simulink model "DemoModel"  (R2019b)
settings: Solver=ode4  StartTime=0.0  StopTime=Inf  FixedStep=0.001  RelTol=1e-3
libraries: fl_lib x42, ElectricalElements x27, nesl_utility x5, simulink x3, ee_lib x2
settings Model: Creator=alfon  LastModifiedBy=Alfonso
settings SFSimCC: CustomCodeUndefinedFunction=UseInterfaceOnly

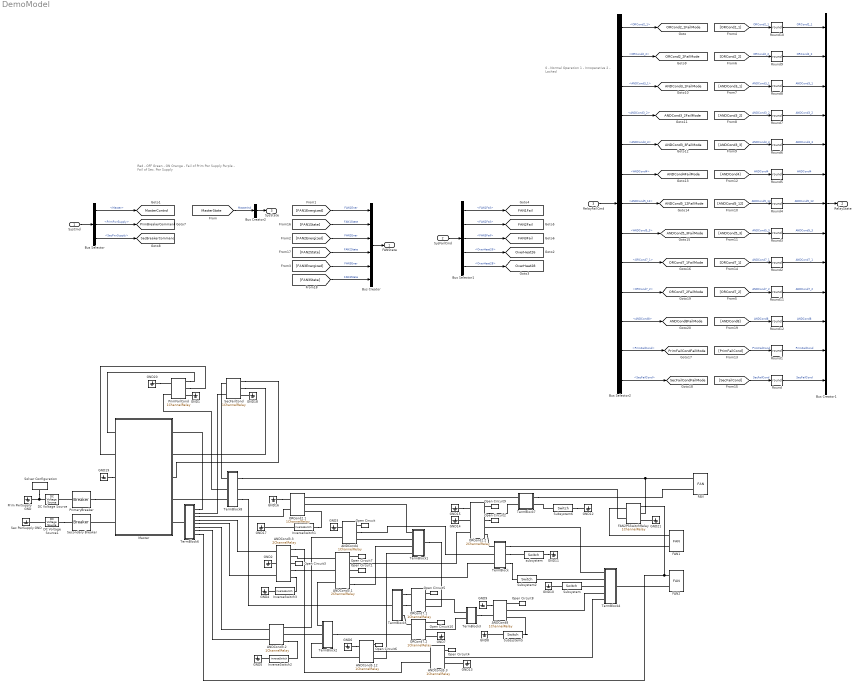
== system DemoModel ==
  note: Red - OFF
      | Green - ON
      | Orange - Fail of Prim Pwr Supply
      | Purple - Fail of Sec. Pwr Supply
  note: 0 - Normal Operation
      | 1 - Innoperative
      | 2 - Lached
  SysCmd : Inport  OutDataTypeStr=Bus: SysCmd  SampleTime=[0.001 0]
  SysFailCmd : Inport  Port=2  OutDataTypeStr=Bus: SysFailCmd  SampleTime=[0.001 0]
  RelayFailCmd : Inport  Port=3  OutDataTypeStr=Bus: RelayFailCmd  SampleTime=[0.001 0]
  ANDCond3.1 : ElectricalElements/Switches/2ChannelRelay  R=100  MinOpVolt=32  MaxOpVolt=22  RelayStateTag=ANDCond3_1  RelayFailModeTag=ANDCond3_1FailMode
  ANDCond3.2 : ElectricalElements/Switches/1ChannelRelay  R=100  MinOpVolt=32  MaxOpVolt=22  RelayStateTag=ANDCond3_2  RelayFailModeTag=ANDCond3_2FailMode
  ANDCond3.3 : ElectricalElements/Switches/2ChannelRelay  R=100  MinOpVolt=32  MaxOpVolt=22  RelayStateTag=ANDCond3_3  RelayFailModeTag=ANDCond3_3FailMode
  ANDCond4 : ElectricalElements/Switches/1ChannelRelay  R=100  MinOpVolt=32  MaxOpVolt=22  RelayStateTag=ANDCond4  RelayFailModeTag=ANDCond4FailMode
  ANDCond5.12 : ElectricalElements/Switches/1ChannelRelay  R=100  MinOpVolt=32  MaxOpVolt=22  RelayStateTag=ANDCond5_12  RelayFailModeTag=ANDCond5_12FailMode
  ANDCond5.3 : ElectricalElements/Switches/1ChannelRelay  R=100  MinOpVolt=32  MaxOpVolt=22  RelayStateTag=ANDCond5_3  RelayFailModeTag=ANDCond5_3FailMode
  ANDCond8 : ElectricalElements/Switches/1ChannelRelay  R=100  MinOpVolt=32  MaxOpVolt=22  RelayStateTag=ANDCond8  RelayFailModeTag=ANDCond8FailMode
  Bus Creator : BusCreator  Inputs=6
  Bus Creator1 : BusCreator  Inputs=13
  Bus Creator2 : BusCreator  Inputs=1
  Bus Selector : BusSelector  OutputSignals=Master,PrimPwrSupply,SecPwrSupply
  Bus Selector1 : BusSelector  OutputSignals=FAN1Fail,FAN2Fail,FAN3Fail,OverHeat26,OverHeat28
  Bus Selector2 : BusSelector  OutputSignals=ORCond2_1,ORCond2_2,ANDCond3_1,ANDCond3_2,ANDCond3_3,ANDCond4,ANDCond5_12,ANDCond5_3,ORCond7_1,ORCond7_2,ANDCond8,PrimFailCond,SecFailCond
  DC Voltage Source : ee_lib/Additional Components/SPICE Sources/DC Voltage Source  DC=28 V
      settings: SourceProductName=Simscape Electrical
  DC Voltage Source1 : ee_lib/Additional Components/SPICE Sources/DC Voltage Source  DC=28 V
      settings: SourceProductName=Simscape Electrical
  FAN : ElectricalElements/FunctionalItems/FAN  FanStatusTag=FAN1State  GotoTag=FAN1Fail  FANNumber=1  FanEnerTag=FAN1Energized
      settings: AttributesFormatString=FAN%<FANNumber>
  FAN1 : ElectricalElements/FunctionalItems/FAN  FanStatusTag=FAN2State  GotoTag=FAN2Fail  FANNumber=2  FanEnerTag=FAN2Energized
      settings: AttributesFormatString=FAN%<FANNumber>
  FAN2 : ElectricalElements/FunctionalItems/FAN  FanStatusTag=FAN3State  GotoTag=FAN3Fail  FANNumber=3  FanEnerTag=FAN3Energized
      settings: AttributesFormatString=FAN%<FANNumber>
  FAN2PSSwitchRelay : ElectricalElements/Switches/1ChannelRelay  R=100  MinOpVolt=32  MaxOpVolt=22  RelayStateTag=A  RelayFailModeTag=A
  GND{1..21} (21 alike) : fl_lib/Electrical/Electrical Elements/Electrical Reference
  InverseSwitch1 : ElectricalElements/Switches/InverseSwitch  SwitchTag=FAN1State
      settings: AttributesFormatString=Inverse %<SwitchTag>
  InverseSwitch2 : ElectricalElements/Switches/InverseSwitch  SwitchTag=FAN2State
      settings: AttributesFormatString=Inverse %<SwitchTag>
  InverseSwitch3 : ElectricalElements/Switches/InverseSwitch  SwitchTag=FAN3State
      settings: AttributesFormatString=Inverse %<SwitchTag>
  Master : Subsystem
  ORCond2.1 : ElectricalElements/Switches/1ChannelRelay  R=100  MinOpVolt=32  MaxOpVolt=22  RelayStateTag=ORCond2_1  RelayFailModeTag=ORCond2_1FailMode
  ORCond2.2 : ElectricalElements/Switches/2ChannelRelay  R=100  MinOpVolt=32  MaxOpVolt=22  RelayStateTag=ORCond2_2  RelayFailModeTag=ORCond2_2FailMode
  ORCond7.1 : ElectricalElements/Switches/1ChannelRelay  R=100  MinOpVolt=32  MaxOpVolt=22  RelayStateTag=ORCond7_1  RelayFailModeTag=ORCond7_1FailMode
  ORCond7.2 : ElectricalElements/Switches/1ChannelRelay  R=100  MinOpVolt=32  MaxOpVolt=22  RelayStateTag=ORCond7_2  RelayFailModeTag=ORCond7_2FailMode
  Open Circuit{,1..10} (11 alike) : fl_lib/Electrical/Electrical Elements/Open Circuit  v_specify=off  v_priority=None  v=0 V  v_nominal_specify=off  v_nominal_unit=V  v_nominal_value=1
      settings: SourceProductName=Simscape  SourceProductBaseCode=SS
  Prim PwrSupply GND : fl_lib/Electrical/Electrical Elements/Electrical Reference
  PrimFailCond : ElectricalElements/Switches/1ChannelRelay  R=100  MinOpVolt=32  MaxOpVolt=22  RelayStateTag=PrimFailCond  RelayFailModeTag=PrimFailCondFailMode
  PrimaryBreaker : ElectricalElements/Switches/Breaker  GotoTag=PrimBreakerCommand
  Round{,1..12} (13 alike) : Rounding  Operator=round
  Sec PwrSupply GND : fl_lib/Electrical/Electrical Elements/Electrical Reference
  SecFailCond : ElectricalElements/Switches/1ChannelRelay  R=100  MinOpVolt=32  MaxOpVolt=22  RelayStateTag=SecFailCond  RelayFailModeTag=SecFailCondFailMode
  Secondary Breaker : ElectricalElements/Switches/Breaker  GotoTag=SecBreakerCommand
  Solver Configuration : nesl_utility/Solver Configuration  PhysicalDomain=network_engine_domain  SubClassName=solver  LeftPortType=input  RightPortType=generic  Tones=[]  Harmonics=[]  SimulateNoise=off  Profile=off  UseLocalSampling=off  EnableSwitchedLinearOptims=on  FrequencyDomain=off  UseCCode=off  RelTol=0.001  AbsTol=1e-06  MinStep=1e-09  ToWorkspace=off  RevertToSquareIcSolve=off  NumHomotopyIterations=100  PhasorMode=off  PhasorModeNumHarmonics=1  DoDC=off  ResidualTolerance=1e-09  UseLocalSolver=off  LocalSolverChoice=NE_BACKWARD_EULER_ADVANCER  LocalSolverSampleTime=0.001  DoFixedCost=off  MaxNonlinIter=3  MaxModeIter=2  LinearAlgebra=auto  EquationFormulation=NE_TIME_EF  DelaysMemoryBudget=1024  AutomaticFiltering=on  FilteringTimeConstant=0.001  PartitionStorageMethod=AS_NEEDED  PartitionMemoryBudget=1024  PartitionMethod=ROBUST
  Subsystem : ElectricalElements/Switches/Switch  SwitchTag=OverHeat28
      settings: AttributesFormatString=%<SwitchTag>
  Subsystem2 : ElectricalElements/Switches/Switch  SwitchTag=OverHeat28
      settings: AttributesFormatString=%<SwitchTag>
  Subsystem5 : ElectricalElements/Switches/Switch  SwitchTag=OverHeat26
      settings: AttributesFormatString=%<SwitchTag>
  Subsystem6 : ElectricalElements/Switches/Switch  SwitchTag=OverHeat28
      settings: AttributesFormatString=%<SwitchTag>
  TermBlock : Subsystem
  TermBlock1 : Subsystem
  TermBlock2 : Subsystem
  TermBlock3 : Subsystem
  TermBlock4 : Subsystem
  TermBlock5 : Subsystem
  TermBlock6 : Subsystem
  TermBlock7 : Subsystem
  TermBlock8 : Subsystem
  subsystem : ElectricalElements/Switches/Switch  SwitchTag=OverHeat26
      settings: AttributesFormatString=%<SwitchTag>
  FANState : Outport  OutDataTypeStr=Bus: FANState  SampleTime=[0.001 0]
  RelayState : Outport  Port=2  OutDataTypeStr=Bus: RelayState  SampleTime=[0.001 0]
  SysState : Outport  Port=3  OutDataTypeStr=Bus: SysState  SampleTime=[0.001 0]
  tag scope: ANDCond3_1FailMode=global, ANDCond3_2FailMode=global, ANDCond3_3FailMode=global, ANDCond4FailMode=global, ANDCond5_12FailMode=global, ANDCond5_3FailMode=global, ANDCond8FailMode=global, FAN1Fail=global, FAN2Fail=global, FAN3Fail=global, MasterControl=global, ORCond2_1FailMode=global, ORCond2_2FailMode=global, ORCond7_1FailMode=global, ORCond7_2FailMode=global, OverHeat26=global, OverHeat28=global, PrimBreakerCommand=global, PrimFailCondFailMode=global, SecBreakerCommand=global, SecFailCondFailMode=global
  wires:
  [MasterState] -> Bus Creator2/1  "MasterInd"
  Bus Selector/1 -> [MasterControl]  "<Master>"
  Bus Selector1/4 -> [OverHeat26]  "<OverHeat26>"
  Bus Selector1/5 -> [OverHeat28]  "<OverHeat28>"
  Bus Selector1/1 -> [FAN1Fail]  "<FAN1Fail>"
  Bus Selector1/2 -> [FAN2Fail]  "<FAN2Fail>"
  Bus Selector1/3 -> [FAN3Fail]  "<FAN3Fail>"
  [FAN1Energized] -> Bus Creator/1  "FAN1Ener"
  [FAN2Energized] -> Bus Creator/3  "FAN2Ener"
  [FAN3Energized] -> Bus Creator/5  "FAN3Ener"
  [ORCond2_1] -> Round10/1  "ORCond2_1"
  [ORCond2_2] -> Round9/1  "ORCond2_2"
  [ANDCond3_1] -> Round8/1  "ANDCond3_1"
  [ANDCond3_2] -> Round7/1  "ANDCond3_2"
  [ANDCond3_3] -> Round6/1  "ANDCond3_3"
  [ANDCond5_12] -> Round4/1  "ANDCond5_12"
  [ANDCond5_3] -> Round3/1  "ANDCond5_3"
  [ANDCond4] -> Round5/1  "ANDCond4"
  [PrimFailCond] -> Round1/1  "PrimFailCond"
  [ORCond7_1] -> Round2/1  "ANDCond7_1"
  [SecFailCond] -> Round/1  "SecFailCond"
  [FAN1State] -> Bus Creator/2  "FAN1State"
  [FAN2State] -> Bus Creator/4  "FAN2State"
  [FAN3State] -> Bus Creator/6  "FAN3State"
  Bus Selector/3 -> [SecBreakerCommand]  "<SecPwrSupply>"
  Bus Selector/2 -> [PrimBreakerCommand]  "<PrimPwrSupply>"
  Bus Selector2/1 -> [ORCond2_1FailMode]  "<ORCond2_1>"
  Bus Selector2/2 -> [ORCond2_2FailMode]  "<ORCond2_2>"
  Bus Selector2/3 -> [ANDCond3_1FailMode]  "<ANDCond3_1>"
  Bus Selector2/4 -> [ANDCond3_2FailMode]  "<ANDCond3_2>"
  Bus Selector2/5 -> [ANDCond3_3FailMode]  "<ANDCond3_3>"
  Bus Selector2/6 -> [ANDCond4FailMode]  "<ANDCond4>"
  Bus Selector2/7 -> [ANDCond5_12FailMode]  "<ANDCond5_12>"
  Bus Selector2/8 -> [ANDCond5_3FailMode]  "<ANDCond5_3>"
  Bus Selector2/9 -> [ORCond7_1FailMode]  "<ORCond7_1>"
  Bus Selector2/12 -> [PrimFailCondFailMode]  "<PrimFailCond>"
  Bus Selector2/13 -> [SecFailCondFailMode]  "<SecFailCond>"
  Round/1 -> Bus Creator1/13  "SecFailCond"
  Round1/1 -> Bus Creator1/12  "PrimFailCond"
  Round2/1 -> Bus Creator1/9  "ANDCond7_1"
  Round3/1 -> Bus Creator1/8  "ANDCond5_3"
  Round4/1 -> Bus Creator1/7  "ANDCond5_12"
  Round5/1 -> Bus Creator1/6  "ANDCond4"
  Round6/1 -> Bus Creator1/5  "ANDCond3_3"
  Round7/1 -> Bus Creator1/4  "ANDCond3_2"
  Round8/1 -> Bus Creator1/3  "ANDCond3_1"
  Round9/1 -> Bus Creator1/2  "ORCond2_2"
  Round10/1 -> Bus Creator1/1  "ORCond2_1"
  Round11/1 -> Bus Creator1/10  "ANDCond7_2"
  Bus Selector2/10 -> [ORCond7_2FailMode]  "<ORCond7_2>"
  [ORCond7_2] -> Round11/1  "ANDCond7_2"
  [ANDCond8] -> Round12/1  "ANDCond8"
  Bus Selector2/11 -> [ANDCond8FailMode]  "<ANDCond8>"
  Round12/1 -> Bus Creator1/11  "ANDCond8"
  Bus Creator/1 -> FANState/1
  Bus Creator1/1 -> RelayState/1
  SysCmd/1 -> Bus Selector/1
  Bus Creator2/1 -> SysState/1
  SysFailCmd/1 -> Bus Selector1/1
  RelayFailCmd/1 -> Bus Selector2/1
  connections:
  DC Voltage Source1/RConn1 -- Sec PwrSupply GND/LConn1
  subsystem/RConn1 -- GND11/LConn1
  Subsystem/RConn1 -- GND10/LConn1
  InverseSwitch1/RConn1 -- GND17/LConn1
  InverseSwitch2/RConn1 -- GND5/LConn1
  InverseSwitch3/RConn1 -- GND4/LConn1
  InverseSwitch1/LConn1 -- ORCond2.1/RConn3
  GND16/LConn1 -- ORCond2.1/LConn1
  ANDCond3.2/RConn3 -- InverseSwitch2/LConn1
  ANDCond3.3/RConn4 -- ANDCond3.1/LConn2
  ANDCond3.3/RConn5 -- InverseSwitch3/LConn1
  Open Circuit1/LConn1 -- ANDCond3.1/RConn3
  DC Voltage Source/RConn1 -- Solver Configuration/RConn1 -- Prim PwrSupply GND/LConn1
  ORCond2.2/RConn3 -- Open Circuit2/LConn1
  ANDCond5.12/RConn2 -- ANDCond5.3/LConn1
  Open Circuit/LConn1 -- ANDCond4/RConn1
  Open Circuit4/LConn1 -- ANDCond5.3/RConn1
  Open Circuit6/LConn1 -- ANDCond5.12/RConn1
  Open Circuit5/LConn1 -- ORCond7.1/RConn1
  ANDCond4/LConn2 -- ANDCond3.2/RConn1
  TermBlock/LConn1 -- ORCond2.2/RConn5
  GND3/LConn1 -- ANDCond4/LConn1
  ORCond2.2/LConn2 -- GND14/LConn1
  GND13/LConn1 -- ANDCond5.3/RConn3
  ANDCond3.3/RConn1 -- ANDCond5.3/LConn2
  Open Circuit3/LConn1 -- ANDCond3.3/RConn3
  Open Circuit7/LConn1 -- ANDCond3.1/RConn1
  GND7/LConn1 -- ORCond7.2/RConn3
  Open Circuit10/LConn1 -- ORCond7.2/RConn1
  Open Circuit8/LConn1 -- ANDCond8/RConn1
  GND9/LConn1 -- ANDCond8/LConn1
  Subsystem5/RConn1 -- GND8/LConn1
  Subsystem5/LConn1 -- ANDCond8/RConn3
  ANDCond3.1/LConn1 -- ANDCond3.3/RConn2
  ORCond2.2/LConn3 -- ANDCond3.1/RConn2
  GND15/LConn1 -- ORCond2.2/LConn1
  Open Circuit9/LConn1 -- ORCond2.2/RConn1
  Subsystem6/RConn1 -- GND12/LConn1
  TermBlock/LConn3 -- ANDCond3.1/RConn4
  TermBlock/RConn3 -- Subsystem2/LConn1
  TermBlock/RConn2 -- subsystem/LConn1
  ANDCond4/RConn2 -- TermBlock/LConn2
  TermBlock/RConn1 -- FAN1/LConn2
  TermBlock1/LConn1 -- ORCond2.1/RConn2
  TermBlock1/LConn2 -- ANDCond4/RConn3
  TermBlock1/RConn1 -- ORCond7.1/RConn3
  TermBlock2/LConn2 -- ANDCond3.2/RConn2
  TermBlock2/LConn1 -- ANDCond3.1/LConn3
  TermBlock2/RConn1 -- ORCond7.2/LConn2
  TermBlock2/LConn3 -- ANDCond5.12/LConn2
  GND6/LConn1 -- ANDCond5.12/LConn1
  TermBlock3/RConn1 -- ANDCond8/LConn2
  TermBlock3/LConn1 -- ORCond7.1/RConn2
  TermBlock3/LConn2 -- ORCond7.2/RConn2
  FAN2/LConn2 -- TermBlock4/RConn1
  TermBlock4/LConn1 -- ORCond2.2/RConn4
  TermBlock4/LConn4 -- ANDCond8/RConn2
  TermBlock4/LConn5 -- ANDCond5.3/RConn2
  TermBlock4/LConn2 -- Subsystem2/RConn1
  TermBlock4/LConn3 -- Subsystem/LConn1
  DC Voltage Source1/LConn1 -- Secondary Breaker/LConn1
  Master/LConn5 -- Secondary Breaker/RConn1
  PrimaryBreaker/RConn1 -- Master/LConn4
  PrimaryBreaker/LConn1 -- DC Voltage Source/LConn1
  GND1/LConn1 -- PrimFailCond/RConn3
  PrimFailCond/RConn2 -- Master/LConn2
  GND18/LConn1 -- SecFailCond/RConn3
  GND20/LConn1 -- PrimFailCond/LConn1
  SecFailCond/RConn2 -- Master/RConn2
  PrimFailCond/RConn1 -- Master/LConn1
  GND19/LConn1 -- Master/LConn3
  ANDCond3.1/RConn5 -- TermBlock1/LConn3
  TermBlock1/LConn4 -- ANDCond5.12/RConn3
  TermBlock5/RConn2 -- ORCond7.1/LConn2
  TermBlock5/RConn1 -- ORCond7.1/LConn1
  ORCond7.2/LConn1 -- TermBlock5/RConn3
  GND2/LConn1 -- ANDCond3.3/LConn2
  SecFailCond/RConn1 -- Master/RConn3
  TermBlock6/LConn1 -- Master/RConn5
  TermBlock6/RConn2 -- SecFailCond/LConn2
  TermBlock6/RConn3 -- ORCond2.1/LConn2
  TermBlock6/RConn4 -- ANDCond3.3/LConn1
  TermBlock6/RConn5 -- ANDCond3.3/LConn3
  TermBlock6/RConn6 -- ANDCond3.2/LConn1
  TermBlock6/RConn7 -- ANDCond3.2/LConn2
  FAN2PSSwitchRelay/LConn2 -- TermBlock8/RConn2
  TermBlock6/RConn1 -- Master/RConn1
  ORCond2.2/RConn2 -- TermBlock7/LConn2
  TermBlock7/LConn1 -- ORCond2.1/RConn1
  Subsystem6/LConn1 -- TermBlock7/RConn2
  TermBlock7/RConn1 -- FAN/LConn2
  TermBlock8/LConn3 -- Master/RConn4
  TermBlock8/LConn2 -- PrimFailCond/LConn2
  TermBlock8/LConn1 -- SecFailCond/LConn1
  TermBlock6/RConn8 -- FAN2PSSwitchRelay/RConn1 -- FAN2/LConn1
  TermBlock8/RConn3 -- TermBlock5/LConn1
  FAN2PSSwitchRelay/LConn1 -- FAN1/LConn1
  GND21/LConn1 -- FAN2PSSwitchRelay/RConn3
  TermBlock8/RConn1 -- FAN2PSSwitchRelay/RConn2 -- FAN/LConn1

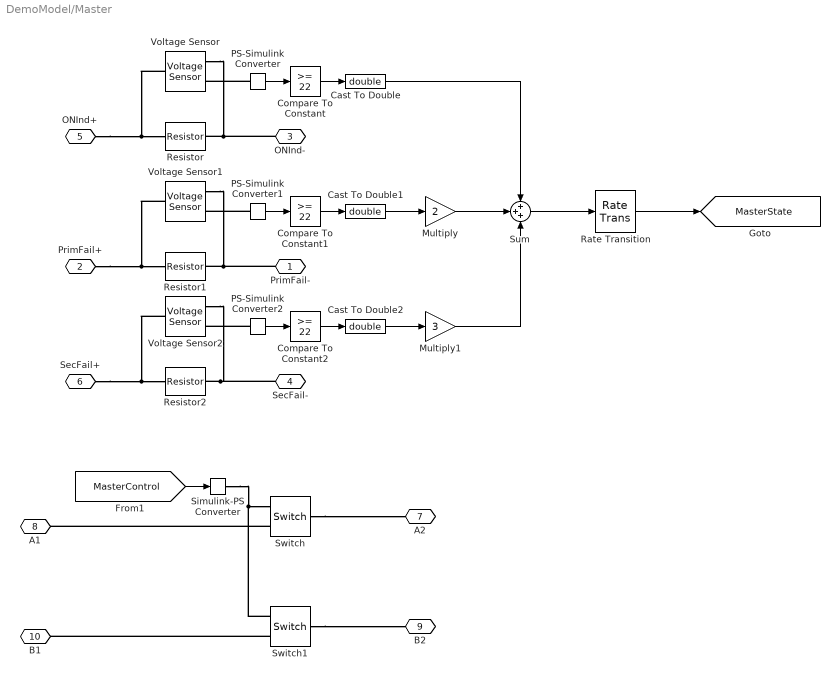
== system DemoModel/Master ==
  Cast To Double : DataTypeConversion  OutDataTypeStr=double
  Cast To Double1 : DataTypeConversion  OutDataTypeStr=double
  Cast To Double2 : DataTypeConversion  OutDataTypeStr=double
  Compare To Constant : simulink/Logic and Bit Operations/Compare To Constant  relop=>=  const=22  OutDataTypeStr=boolean
  Compare To Constant1 : simulink/Logic and Bit Operations/Compare To Constant  relop=>=  const=22  OutDataTypeStr=boolean
  Compare To Constant2 : simulink/Logic and Bit Operations/Compare To Constant  relop=>=  const=22  OutDataTypeStr=boolean
  Multiply : Gain  Gain=2
  Multiply1 : Gain  Gain=3
  PS-Simulink Converter : nesl_utility/PS-Simulink Converter  PhysicalDomain=network_engine_domain  SubClassName=ps_output  LeftPortType=input  RightPortType=output  PseudoPeriodic=off  Frequencies=[]  Unit=1  AffineConversion=off
  PS-Simulink Converter1 : nesl_utility/PS-Simulink Converter  PhysicalDomain=network_engine_domain  SubClassName=ps_output  LeftPortType=input  RightPortType=output  PseudoPeriodic=off  Frequencies=[]  Unit=1  AffineConversion=off
  PS-Simulink Converter2 : nesl_utility/PS-Simulink Converter  PhysicalDomain=network_engine_domain  SubClassName=ps_output  LeftPortType=input  RightPortType=output  PseudoPeriodic=off  Frequencies=[]  Unit=1  AffineConversion=off
  Rate Transition : RateTransition  OutPortSampleTime=[0.001 0]
  Resistor : fl_lib/Electrical/Electrical Elements/Resistor  R=100 Ohm  i_specify=off  i_priority=None  i=0 A  i_nominal_specify=off  i_nominal_unit=A  i_nominal_value=1  v_specify=off  v_priority=None  v=0 V  v_nominal_specify=off  v_nominal_unit=V  v_nominal_value=1
  Resistor1 : fl_lib/Electrical/Electrical Elements/Resistor  R=100 Ohm  i_specify=off  i_priority=None  i=0 A  i_nominal_specify=off  i_nominal_unit=A  i_nominal_value=1  v_specify=off  v_priority=None  v=0 V  v_nominal_specify=off  v_nominal_unit=V  v_nominal_value=1
  Resistor2 : fl_lib/Electrical/Electrical Elements/Resistor  R=100 Ohm  i_specify=off  i_priority=None  i=0 A  i_nominal_specify=off  i_nominal_unit=A  i_nominal_value=1  v_specify=off  v_priority=None  v=0 V  v_nominal_specify=off  v_nominal_unit=V  v_nominal_value=1
  Simulink-PS Converter : nesl_utility/Simulink-PS Converter  PhysicalDomain=network_engine_domain  SubClassName=ps_input  LeftPortType=input  RightPortType=output  PseudoPeriodic=off  Frequencies=[]  NoiseDistribution=none  NoiseParameters=[]  Unit=1  AffineConversion=off  FilteringAndDerivatives=provide  SimscapeFilterOrder=1  InputFilterTimeConstant=0.001  UdotUserProvided=0
  Sum : Sum  Inputs=+++
  Switch : fl_lib/Electrical/Electrical Elements/Switch  R_closed=0.01 Ohm  G_open=1e-8 1/Ohm  Threshold=0.5  i_specify=off  i_priority=None  i=0 A  i_nominal_specify=off  i_nominal_unit=A  i_nominal_value=1  v_specify=off  v_priority=None  v=0 V  v_nominal_specify=off  v_nominal_unit=V  v_nominal_value=1
      settings: SourceProductName=Simscape
  Switch1 : fl_lib/Electrical/Electrical Elements/Switch  R_closed=0.01 Ohm  G_open=1e-8 1/Ohm  Threshold=0.5  i_specify=off  i_priority=None  i=0 A  i_nominal_specify=off  i_nominal_unit=A  i_nominal_value=1  v_specify=off  v_priority=None  v=0 V  v_nominal_specify=off  v_nominal_unit=V  v_nominal_value=1
      settings: SourceProductName=Simscape
  Voltage Sensor : fl_lib/Electrical/Electrical Sensors/Voltage Sensor
  Voltage Sensor1 : fl_lib/Electrical/Electrical Sensors/Voltage Sensor
  Voltage Sensor2 : fl_lib/Electrical/Electrical Sensors/Voltage Sensor
  PrimFail- : PMIOPort  Side=Left
  PrimFail+ : PMIOPort  Port=2  Side=Right
  ONInd- : PMIOPort  Port=3  Side=Left
  SecFail- : PMIOPort  Port=4  Side=Left
  ONInd+ : PMIOPort  Port=5  Side=Right
  SecFail+ : PMIOPort  Port=6  Side=Right
  A2 : PMIOPort  Port=7  Side=Right
  A1 : PMIOPort  Port=8  Side=Left
  B2 : PMIOPort  Port=9  Side=Right
  B1 : PMIOPort  Port=10  Side=Left
  tag scope: MasterState=global
  wires:
  Compare To Constant/1 -> Cast To Double/1
  PS-Simulink Converter/1 -> Compare To Constant/1
  [MasterControl] -> Simulink-PS Converter/1
  PS-Simulink Converter1/1 -> Compare To Constant1/1
  Cast To Double1/1 -> Multiply/1
  Compare To Constant1/1 -> Cast To Double1/1
  Sum/1 -> Rate Transition/1
  Cast To Double/1 -> Sum/1
  Multiply/1 -> Sum/2
  Multiply1/1 -> Sum/3
  Compare To Constant2/1 -> Cast To Double2/1
  Cast To Double2/1 -> Multiply1/1
  PS-Simulink Converter2/1 -> Compare To Constant2/1
  Rate Transition/1 -> [MasterState]
  connections:
  Simulink-PS Converter/RConn1 -- Switch1/RConn1 -- Switch/RConn1
  Voltage Sensor/RConn2 -- ONInd-/RConn1 -- Resistor/RConn1
  Voltage Sensor/LConn1 -- Resistor/LConn1 -- ONInd+/RConn1
  PS-Simulink Converter/LConn1 -- Voltage Sensor/RConn1
  Switch1/RConn2 -- B1/RConn1
  Switch/RConn2 -- A1/RConn1
  Switch1/LConn1 -- B2/RConn1
  Switch/LConn1 -- A2/RConn1
  Voltage Sensor1/RConn2 -- Resistor1/RConn1 -- PrimFail-/RConn1
  Voltage Sensor1/LConn1 -- PrimFail+/RConn1 -- Resistor1/LConn1
  PS-Simulink Converter1/LConn1 -- Voltage Sensor1/RConn1
  Resistor2/RConn1 -- Voltage Sensor2/RConn2 -- SecFail-/RConn1
  SecFail+/RConn1 -- Voltage Sensor2/LConn1 -- Resistor2/LConn1
  PS-Simulink Converter2/LConn1 -- Voltage Sensor2/RConn1

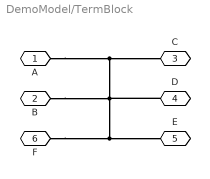
== system DemoModel/TermBlock ==
  A : PMIOPort  Side=Left
  B : PMIOPort  Port=2  Side=Left
  C : PMIOPort  Port=3  Side=Right
  D : PMIOPort  Port=4  Side=Right
  E : PMIOPort  Port=5  Side=Right
  F : PMIOPort  Port=6  Side=Left
  connections:
  A/RConn1 -- F/RConn1 -- E/RConn1 -- D/RConn1 -- B/RConn1 -- C/RConn1

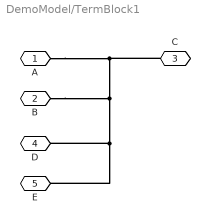
== system DemoModel/TermBlock1 ==
  A : PMIOPort  Side=Left
  B : PMIOPort  Port=2  Side=Left
  C : PMIOPort  Port=3  Side=Right
  D : PMIOPort  Port=4  Side=Left
  E : PMIOPort  Port=5  Side=Left
  connections:
  D/RConn1 -- C/RConn1 -- A/RConn1 -- B/RConn1 -- E/RConn1

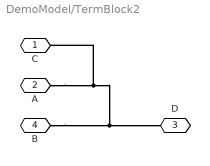
== system DemoModel/TermBlock2 ==
  C : PMIOPort  Side=Left
  A : PMIOPort  Port=2  Side=Left
  D : PMIOPort  Port=3  Side=Right
  B : PMIOPort  Port=4  Side=Left
  connections:
  C/RConn1 -- B/RConn1 -- D/RConn1 -- A/RConn1

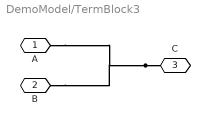
== system DemoModel/TermBlock3 ==
  A : PMIOPort  Side=Left
  B : PMIOPort  Port=2  Side=Left
  C : PMIOPort  Port=3  Side=Right
  connections:
  C/RConn1 -- A/RConn1 -- B/RConn1

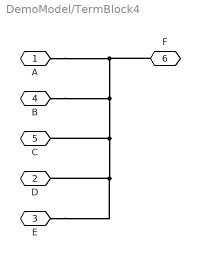
== system DemoModel/TermBlock4 ==
  A : PMIOPort  Side=Left
  D : PMIOPort  Port=2  Side=Left
  E : PMIOPort  Port=3  Side=Left
  B : PMIOPort  Port=4  Side=Left
  C : PMIOPort  Port=5  Side=Left
  F : PMIOPort  Port=6  Side=Right
  connections:
  C/RConn1 -- F/RConn1 -- A/RConn1 -- B/RConn1 -- D/RConn1 -- E/RConn1

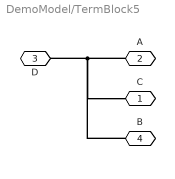
== system DemoModel/TermBlock5 ==
  C : PMIOPort  Side=Right
  A : PMIOPort  Port=2  Side=Right
  D : PMIOPort  Port=3  Side=Left
  B : PMIOPort  Port=4  Side=Right
  connections:
  A/RConn1 -- B/RConn1 -- C/RConn1 -- D/RConn1

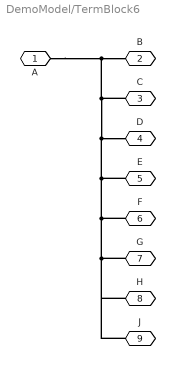
== system DemoModel/TermBlock6 ==
  A : PMIOPort  Side=Left
  B : PMIOPort  Port=2  Side=Right
  C : PMIOPort  Port=3  Side=Right
  D : PMIOPort  Port=4  Side=Right
  E : PMIOPort  Port=5  Side=Right
  F : PMIOPort  Port=6  Side=Right
  G : PMIOPort  Port=7  Side=Right
  H : PMIOPort  Port=8  Side=Right
  J : PMIOPort  Port=9  Side=Right
  connections:
  C/RConn1 -- J/RConn1 -- H/RConn1 -- G/RConn1 -- F/RConn1 -- E/RConn1 -- D/RConn1 -- B/RConn1 -- A/RConn1

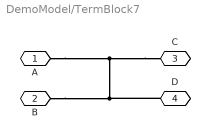
== system DemoModel/TermBlock7 ==
  A : PMIOPort  Side=Left
  B : PMIOPort  Port=2  Side=Left
  C : PMIOPort  Port=3  Side=Right
  D : PMIOPort  Port=4  Side=Right
  connections:
  C/RConn1 -- B/RConn1 -- D/RConn1 -- A/RConn1

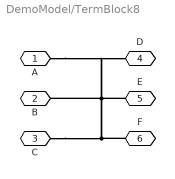
== system DemoModel/TermBlock8 ==
  A : PMIOPort  Side=Left
  B : PMIOPort  Port=2  Side=Left
  C : PMIOPort  Port=3  Side=Left
  D : PMIOPort  Port=4  Side=Right
  E : PMIOPort  Port=5  Side=Right
  F : PMIOPort  Port=6  Side=Right
  connections:
  F/RConn1 -- E/RConn1 -- A/RConn1 -- D/RConn1 -- B/RConn1 -- C/RConn1
